simulink model "ip_ctr_test"  (Simulink 7.3)
settings: Solver=ode45  StartTime=0.0  StopTime=10.0  RelTol=1e-3
libraries: xps_library x8, xbsIndex_r4 x3
settings Model: Creator=tfiliba  LastModifiedBy=tfiliba

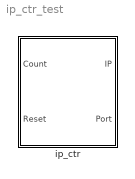
== system ip_ctr_test ==
  ip_ctr : Subsystem  mask(ip_ctr){numcomputers=4}
      mask prompts: numcomputers "Num IPs (Must be power of 2)"
      mask init:
      | ip_ctr_init(gcb,...
      |     'numcomputers',numcomputers)
      settings: AttributesFormatString=IPs=4

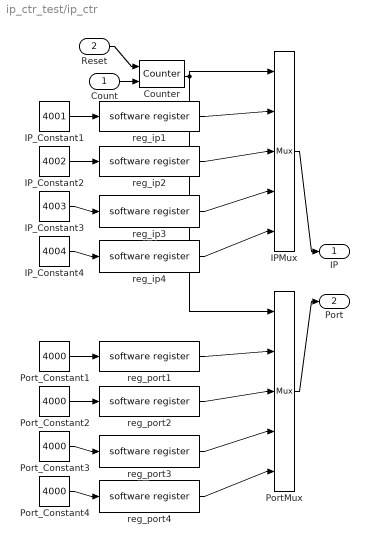
== system ip_ctr_test/ip_ctr ==
  Count : Inport
  Reset : Inport  Port=2  OutDataType=sfix(16)  OutScaling=2^0
  Counter : xbsIndex_r4/Counter  cnt_type=Free Running  cnt_to=Inf  operation=Up  start_count=0  cnt_by_val=1  arith_type=Unsigned  n_bits=2  bin_pt=0  load_pin=off  rst=on  en=on  explicit_period=on  period=1  dbl_ovrd=off  use_behavioral_HDL=off  implementation=Fabric  block_type=counter
      settings: block_version=11.4
  IPMux : xbsIndex_r4/Mux  inputs=4  en=off  latency=3  precision=Full  arith_type=Unsigned  n_bits=16  bin_pt=14  quantization=Truncate  overflow=Wrap  dbl_ovrd=off  block_type=mux
      settings: block_version=11.4
  IP_Constant1 : Constant  Value=4001  OutDataType=sfix(16)  OutScaling=2^0
  IP_Constant2 : Constant  Value=4002  OutDataType=sfix(16)  OutScaling=2^0
  IP_Constant3 : Constant  Value=4003  OutDataType=fixdt(1, 16)  OutScaling=2^0
  IP_Constant4 : Constant  Value=4004  OutDataType=fixdt(1, 16)  OutScaling=2^0
  PortMux : xbsIndex_r4/Mux  inputs=4  en=off  latency=3  precision=Full  arith_type=Unsigned  n_bits=16  bin_pt=14  quantization=Truncate  overflow=Wrap  dbl_ovrd=off  block_type=mux
      settings: block_version=11.4
  Port_Constant1 : Constant  Value=4000  OutDataType=sfix(16)  OutScaling=2^0
  Port_Constant2 : Constant  Value=4000  OutDataType=sfix(16)  OutScaling=2^0
  Port_Constant3 : Constant  Value=4000  OutDataType=fixdt(1, 16)  OutScaling=2^0
  Port_Constant4 : Constant  Value=4000  OutDataType=fixdt(1, 16)  OutScaling=2^0
  reg_ip1 : xps_library/software register  Tag=xps:sw_reg  SystemSampleTime=-1  io_dir=From Processor  arith_type=Unsigned  bitwidth=32  bin_pt=0  sample_period=1  gw_name=untitled_ip_ctr_reg_ip1_user_data_out
      link override pasp_16i16c128s_pasp_dist_gbe_ip_ctr_reg_ip1_user_data_out: arith_type=Unsigned  n_bits=32  bin_pt=0  period=1
  reg_ip2 : xps_library/software register  Tag=xps:sw_reg  SystemSampleTime=-1  io_dir=From Processor  arith_type=Unsigned  bitwidth=32  bin_pt=0  sample_period=1  gw_name=untitled_ip_ctr_reg_ip2_user_data_out
      link override pasp_16i16c128s_pasp_dist_gbe_ip_ctr_reg_ip2_user_data_out: arith_type=Unsigned  n_bits=32  bin_pt=0  period=1
  reg_ip3 : xps_library/software register  Tag=xps:sw_reg  SystemSampleTime=-1  io_dir=From Processor  arith_type=Unsigned  bitwidth=32  bin_pt=0  sample_period=1  gw_name=untitled_ip_ctr_reg_ip3_user_data_out
  reg_ip4 : xps_library/software register  Tag=xps:sw_reg  SystemSampleTime=-1  io_dir=From Processor  arith_type=Unsigned  bitwidth=32  bin_pt=0  sample_period=1  gw_name=untitled_ip_ctr_reg_ip4_user_data_out
  reg_port1 : xps_library/software register  Tag=xps:sw_reg  SystemSampleTime=-1  io_dir=From Processor  arith_type=Unsigned  bitwidth=32  bin_pt=0  sample_period=1  gw_name=untitled_ip_ctr_reg_port1_user_data_out
      link override pasp_16i16c128s_pasp_dist_gbe_ip_ctr_reg_port1_user_data_out: arith_type=Unsigned  n_bits=32  bin_pt=0  period=1
  reg_port2 : xps_library/software register  Tag=xps:sw_reg  SystemSampleTime=-1  io_dir=From Processor  arith_type=Unsigned  bitwidth=32  bin_pt=0  sample_period=1  gw_name=untitled_ip_ctr_reg_port2_user_data_out
      link override pasp_16i16c128s_pasp_dist_gbe_ip_ctr_reg_port2_user_data_out: arith_type=Unsigned  n_bits=32  bin_pt=0  period=1
  reg_port3 : xps_library/software register  Tag=xps:sw_reg  SystemSampleTime=-1  io_dir=From Processor  arith_type=Unsigned  bitwidth=32  bin_pt=0  sample_period=1  gw_name=untitled_ip_ctr_reg_port3_user_data_out
  reg_port4 : xps_library/software register  Tag=xps:sw_reg  SystemSampleTime=-1  io_dir=From Processor  arith_type=Unsigned  bitwidth=32  bin_pt=0  sample_period=1  gw_name=untitled_ip_ctr_reg_port4_user_data_out
  IP : Outport
  Port : Outport  Port=2
  wires:
  Reset/1 -> Counter/1
  Count/1 -> Counter/2
  Counter/1 -> IPMux/1, PortMux/1
  IPMux/1 -> IP/1
  PortMux/1 -> Port/1
  IP_Constant1/1 -> reg_ip1/1
  reg_ip1/1 -> IPMux/2
  Port_Constant1/1 -> reg_port1/1
  reg_port1/1 -> PortMux/2
  IP_Constant2/1 -> reg_ip2/1
  reg_ip2/1 -> IPMux/3
  Port_Constant2/1 -> reg_port2/1
  reg_port2/1 -> PortMux/3
  IP_Constant3/1 -> reg_ip3/1
  reg_ip3/1 -> IPMux/4
  Port_Constant3/1 -> reg_port3/1
  reg_port3/1 -> PortMux/4
  IP_Constant4/1 -> reg_ip4/1
  reg_ip4/1 -> IPMux/5
  Port_Constant4/1 -> reg_port4/1
  reg_port4/1 -> PortMux/5
